simulink model "slip_calc"  (R2024a)
settings: Solver=VariableStepAuto  StartTime=0.0  StopTime=10.0  RelTol=1e-3
settings Model: Creator=fjmo  LastModifiedBy=fjmo

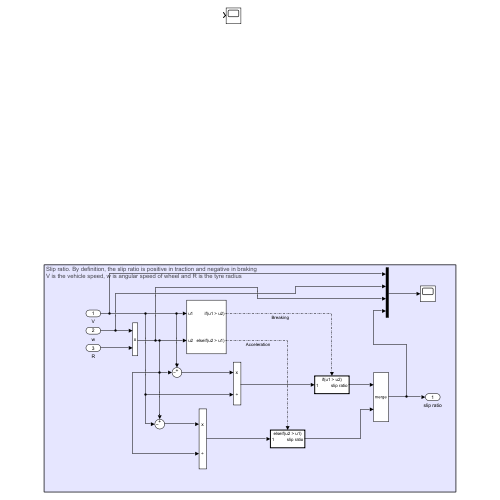
[thumbnail: Simulink's stored preview of the top-level diagram]
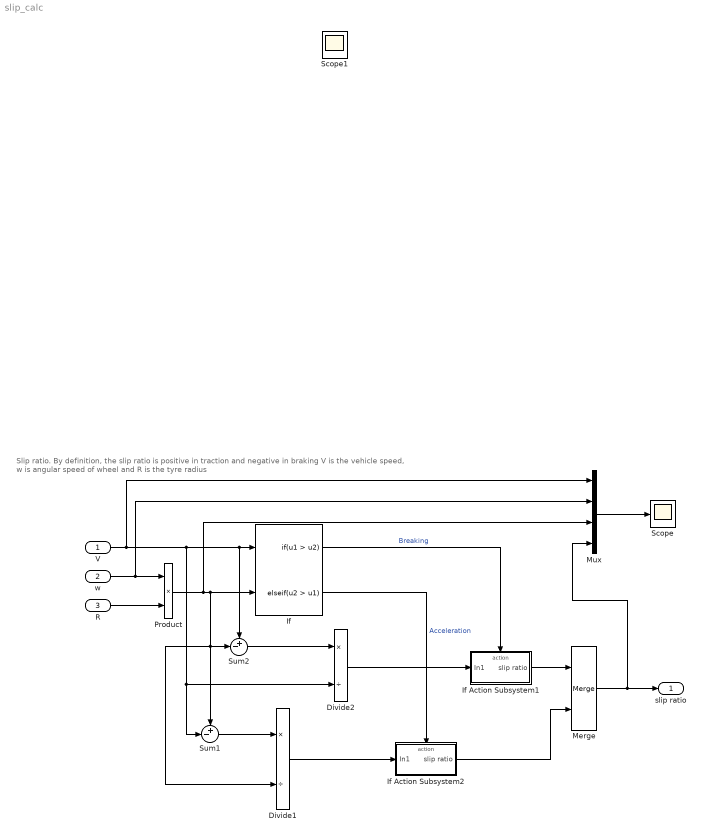
== system slip_calc ==
  note: Slip ratio. By definition, the slip ratio is positive in traction and negative in braking
      | V is the vehicle speed, w is angular speed of wheel and R is the tyre radius
  V : Inport
  w : Inport  Port=2
  R : Inport  Port=3
  Divide1 : Product  Inputs=*/
  Divide2 : Product  Inputs=*/
  If : If  NumInputs=2  IfExpression=u1 > u2  ElseIfExpressions=u2 > u1  ShowElse=off
  If Action Subsystem1 : Subsystem  TreatAsAtomicUnit=on
  If Action Subsystem2 : Subsystem  TreatAsAtomicUnit=on
  Merge : Merge
  Mux : Mux
  Product : Product
  Scope : Scope
  Scope1 : Scope
  Sum1 : Sum  Inputs=+-|
  Sum2 : Sum  Inputs=+-|
  slip ratio : Outport
  wires:
  If/1 -> If Action Subsystem1/Action  "Breaking"
  If/2 -> If Action Subsystem2/Action  "Acceleration"
  Divide1/1 -> If Action Subsystem2/1(In1)
  Divide2/1 -> If Action Subsystem1/1(In1)
  If Action Subsystem1/1(slip ratio) -> Merge/1
  If Action Subsystem2/1(slip ratio) -> Merge/2
  Merge/1 -> Mux/4, slip ratio/1
  Product/1 -> Mux/3, If/2, Divide1/2, Sum1/1, Sum2/2
  w/1 -> Mux/2, Product/1
  V/1 -> Mux/1, Sum2/1, If/1, Sum1/2, Divide2/2
  R/1 -> Product/2
  Sum2/1 -> Divide2/1
  Sum1/1 -> Divide1/1
  Mux/1 -> Scope/1

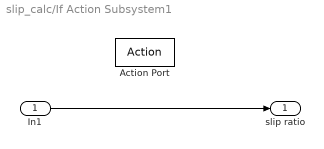
== system slip_calc/If Action Subsystem1 ==
  In1 : Inport
  Action Port : ActionPort  ActionPortLabel=if(u1 > u2)
  slip ratio : Outport
  wires:
  In1/1 -> slip ratio/1

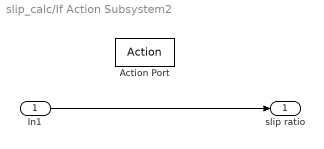
== system slip_calc/If Action Subsystem2 ==
  In1 : Inport
  Action Port : ActionPort  ActionPortLabel=elseif(u2 > u1)
  slip ratio : Outport
  wires:
  In1/1 -> slip ratio/1
